simulink model "rv9level"  (R2017a)
settings: Solver=VariableStepAuto  StartTime=0.0  StopTime=0.3  MaxStep=1e-4  RelTol=1e-3
libraries: powerlib x48, simulink x4, commsynccomp2 x1, dsparch4 x1, powerlib_meascontrol x1
settings Model: Creator=Bilal Ahmed  LastModifiedBy=Bilal Ahmed

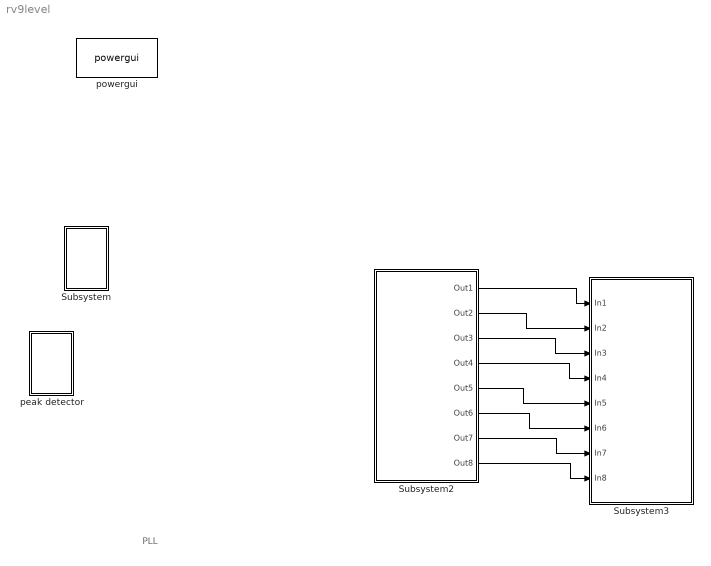
== system rv9level ==
  note: PLL
  Subsystem : Subsystem
  Subsystem2 : Subsystem
  Subsystem3 : Subsystem
  peak detector : Subsystem
  powergui : powerlib/powergui  Priority=1  SimulationMode=Continuous  SampleTime=1e-3  frequency=60  Iterations=50  frequencyindice=0  Pbase=100e6  ErrMax=1e-4  UnitsV=kV  UnitsW=MW  buscounter=0  FunctionMessages=off  echomessages=off  EnableUseOfTLC=off  CurrentSourceSwitches=off  DisableSnubberDevices=off  DisableRonSwitches=off  DisableVfSwitches=off  DisplayEquations=off  SolverType=Tustin/Backward Euler (TBE)  Interpol=off  ExternalGateDelay=off  methode=off  Ts=100  x0status=blocks  SPID=on  SwTol=0  HookPort=off  RestoreLinks=warning  ResistiveCurrentMeasurement=off  Frange=[0:2:500]  Ylog=off  Xlog=on  ShowGrid=off  save=off  variable=ZData  structure=0  ZoomFFT=off  StartTime=0.0  cycles=1  DisplayStyle=1  fundamental=60  FreqAxis=off  MaxFrequency=1000  frequencyindicesteady=1  RmsSteady=1  display=off
  wires:
  Subsystem2/3(Out3) -> Subsystem3/3(In3)
  Subsystem2/6(Out6) -> Subsystem3/6(In6)
  Subsystem2/5(Out5) -> Subsystem3/5(In5)
  Subsystem2/4(Out4) -> Subsystem3/4(In4)
  Subsystem2/2(Out2) -> Subsystem3/2(In2)
  Subsystem2/1(Out1) -> Subsystem3/1(In1)
  Subsystem2/7(Out7) -> Subsystem3/7(In7)
  Subsystem2/8(Out8) -> Subsystem3/8(In8)

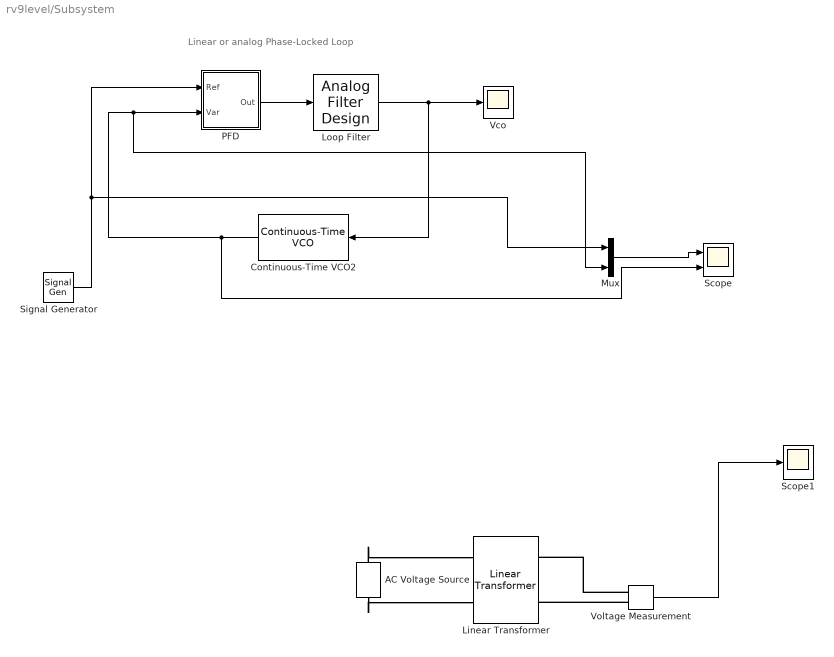
== system rv9level/Subsystem ==
  note: Linear or analog Phase-Locked Loop
  AC Voltage Source : powerlib/Electrical Sources/AC Voltage Source  Amplitude=154  Phase=0  Frequency=50  SampleTime=0  Measurements=None  BusType=PV  Pref=10e3  Qref=0  Qmin=-inf  Qmax=+inf
  Continuous-Time VCO2 : commsynccomp2/Continuous-Time VCO  Ac=2  Fc=46  Kc=8  Ph=0
      settings: SourceProductName=Communications System Toolbox  SourceProductBaseCode=CM
  Linear Transformer : powerlib/Elements/Linear Transformer  UNITS=SI  NominalPower=[ 1100 50 ]  winding1=[220 0 0]  winding2=[7 0 0]  ThreeWindings=off  winding3=[3.15e+05 7.8765e+07 26602]  RmLm=[Inf Inf]  Measurements=None  DataType=on
  Loop Filter : dsparch4/Analog Filter Design  method=Butterworth  filttype=Lowpass  N=5  Wlo=50*2*pi  Whi=80  Rp=1  Rs=180
  Mux : Mux  Inputs=2
  PFD : Subsystem
  Scope : Scope  NumInputPorts=2
  Scope1 : Scope
  Signal Generator : SignalGenerator  Amplitude=2  Frequency=2*pi*50  Units=rad/sec
  Vco : Scope
  Voltage Measurement : powerlib/Measurements/Voltage Measurement  PhasorSimulation=off  OutputType=Complex  PSBequivalent=0
  wires:
  Loop Filter/1 -> Vco/1, Continuous-Time VCO2/1
  PFD/1(Out) -> Loop Filter/1
  Mux/1 -> Scope/1
  Continuous-Time VCO2/1 -> Scope/2, Mux/2, PFD/2(Var)
  Signal Generator/1 -> Mux/1, PFD/1(Ref)
  Voltage Measurement/1 -> Scope1/1
  connections:
  AC Voltage Source/RConn1 -- Linear Transformer/LConn1
  AC Voltage Source/LConn1 -- Linear Transformer/LConn2
  Voltage Measurement/LConn1 -- Linear Transformer/RConn1
  Voltage Measurement/LConn2 -- Linear Transformer/RConn2

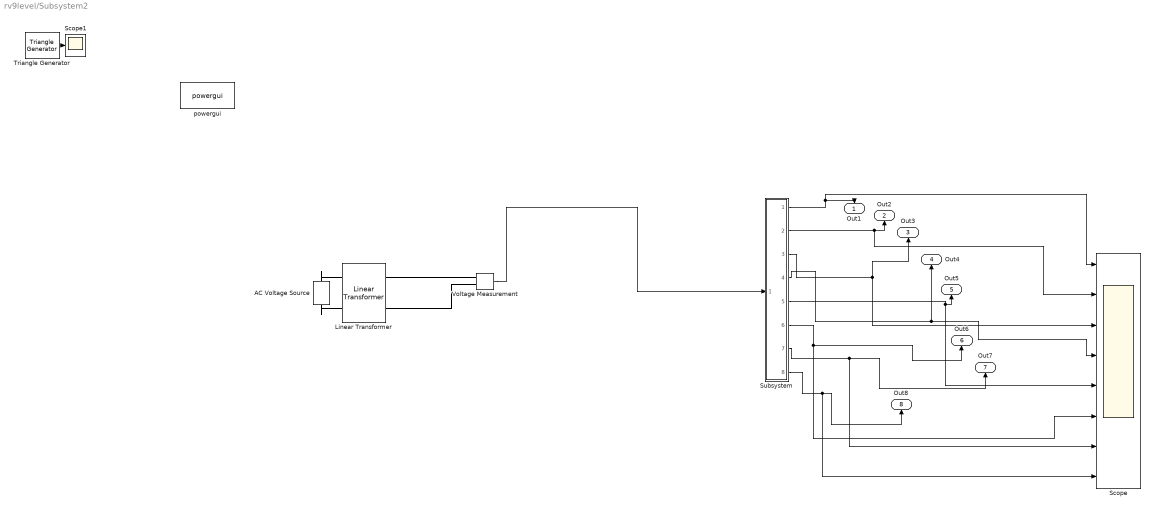
== system rv9level/Subsystem2 ==
  AC Voltage Source : powerlib/Electrical Sources/AC Voltage Source  Amplitude=220  Phase=0  Frequency=50  SampleTime=0  Measurements=None  BusType=PV  Pref=10e3  Qref=0  Qmin=-inf  Qmax=+inf
  Linear Transformer : powerlib/Elements/Linear Transformer  UNITS=pu  NominalPower=[1100 50 ]  winding1=[154 0 0]  winding2=[3.5 0 0]  ThreeWindings=off  winding3=[3.15e+05 9.68e-09 3.2267e-07]  RmLm=[Inf Inf]  Measurements=None  DataType=off
  Scope : Scope  NumInputPorts=8
  Scope1 : Scope
  Subsystem : Subsystem
  Triangle Generator : powerlib_meascontrol/Pulse & Signal Generators/Triangle Generator  Freq=1e6  Phase=0  Ts=0
  Voltage Measurement : powerlib/Measurements/Voltage Measurement  PhasorSimulation=off  OutputType=Complex  PSBequivalent=0
  powergui : powerlib/powergui  Priority=1  SimulationMode=Continuous  SampleTime=50e-6  frequency=60  Iterations=50  frequencyindice=60  Pbase=100e6  ErrMax=1e-4  UnitsV=kV  UnitsW=MW  buscounter=0  FunctionMessages=off  echomessages=off  EnableUseOfTLC=off  CurrentSourceSwitches=off  DisableSnubberDevices=off  DisableRonSwitches=off  DisableVfSwitches=off  DisplayEquations=off  SolverType=Tustin/Backward Euler (TBE)  Interpol=off  ExternalGateDelay=off  methode=off  Ts=100  x0status=blocks  SPID=on  SwTol=0  HookPort=off  RestoreLinks=warning  ResistiveCurrentMeasurement=off  Frange=[0:2:500]  Ylog=off  Xlog=on  ShowGrid=off  save=off  variable=ZData  structure=0  ZoomFFT=off  StartTime=0.0  cycles=1  DisplayStyle=1  fundamental=60  FreqAxis=off  MaxFrequency=1000  frequencyindicesteady=1  RmsSteady=1  display=off
  Out1 : Outport
  Out2 : Outport  Port=2
  Out3 : Outport  Port=3
  Out4 : Outport  Port=4
  Out5 : Outport  Port=5
  Out6 : Outport  Port=6
  Out7 : Outport  Port=7
  Out8 : Outport  Port=8
  wires:
  Voltage Measurement/1 -> Subsystem/1(In1)
  Triangle Generator/1 -> Scope1/1
  Subsystem/1(Out1) -> Scope/1, Out1/1
  Subsystem/2(Out2) -> Scope/2, Out2/1
  Subsystem/3(Out3) -> Out3/1, Scope/3
  Subsystem/6(Out4) -> Scope/6, Out6/1
  Subsystem/4(Out5) -> Scope/4, Out4/1
  Subsystem/5(Out6) -> Scope/5, Out5/1
  Subsystem/8(Out8) -> Scope/8, Out8/1
  Subsystem/7(Out7) -> Scope/7, Out7/1
  connections:
  Linear Transformer/RConn2 -- Voltage Measurement/LConn2
  AC Voltage Source/LConn1 -- Linear Transformer/LConn2
  Voltage Measurement/LConn1 -- Linear Transformer/RConn1
  AC Voltage Source/RConn1 -- Linear Transformer/LConn1

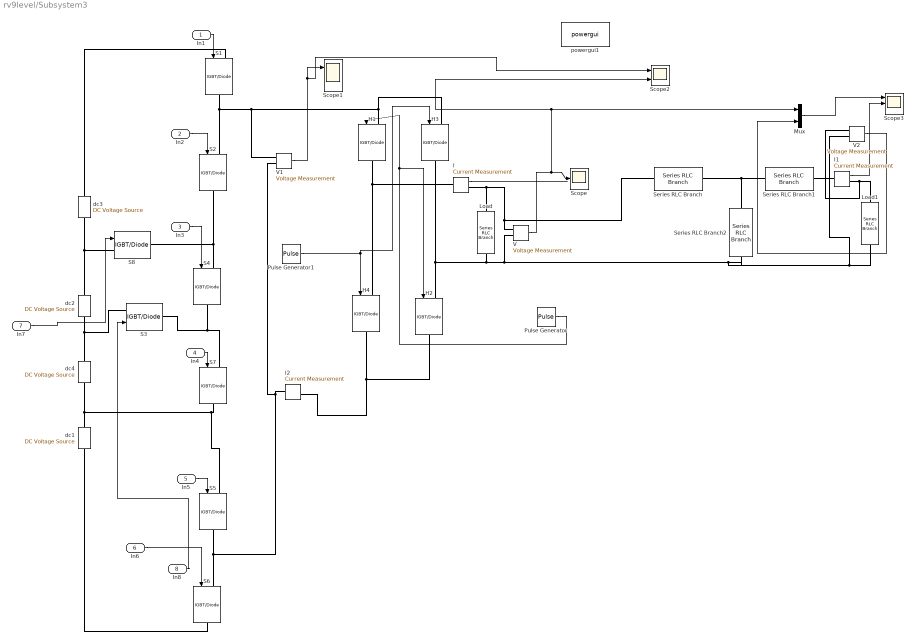
== system rv9level/Subsystem3 ==
  In1 : Inport
  In2 : Inport  Port=2
  In3 : Inport  Port=3
  In4 : Inport  Port=4
  In5 : Inport  Port=5
  In6 : Inport  Port=6
  In7 : Inport  Port=7
  In8 : Inport  Port=8
  H{1..4} (4 alike) : powerlib/Power Electronics/IGBT//Diode  Ron=1e-3  Rs=1e5  Cs=inf  Measurements=off
  I : powerlib/Measurements/Current Measurement  PhasorSimulation=off  OutputType=Complex  PSBequivalent=0
  I1 : powerlib/Measurements/Current Measurement  PhasorSimulation=off  OutputType=Complex  PSBequivalent=0
  I2 : powerlib/Measurements/Current Measurement  PhasorSimulation=off  OutputType=Complex  PSBequivalent=0
  Load : powerlib/Elements/Series RLC Branch  LConnTagsString=__new0  RConnTagsString=__new0  BranchType=R  Resistance=10  Inductance=1e-3  SetiL0=off  InitialCurrent=0  Capacitance=1e-6  Setx0=off  InitialVoltage=0  Measurements=None
  Load1 : powerlib/Elements/Series RLC Branch  LConnTagsString=__new0  RConnTagsString=__new0  BranchType=R  Resistance=10  Inductance=1e-3  SetiL0=off  InitialCurrent=0  Capacitance=1e-6  Setx0=off  InitialVoltage=0  Measurements=None
  Mux : Mux  Inputs=2
  Pulse Generator : DiscretePulseGenerator  PulseType=Time based  Period=0.02  PulseWidth=50
  Pulse Generator1 : DiscretePulseGenerator  PulseType=Time based  Period=0.02  PulseWidth=50  PhaseDelay=.01
  S{1..8} (8 alike) : powerlib/Power Electronics/IGBT//Diode  Ron=1e-3  Rs=1e5  Cs=inf  Measurements=off
  Scope : Scope
  Scope1 : Scope  NumInputPorts=2
  Scope2 : Scope  NumInputPorts=2
  Scope3 : Scope  NumInputPorts=3
  Series RLC Branch : powerlib/Elements/Series RLC Branch  LConnTagsString=__new0  RConnTagsString=__new0  BranchType=L  Resistance=1  Inductance=1e-3  SetiL0=off  InitialCurrent=0  Capacitance=1e-6  Setx0=off  InitialVoltage=0  Measurements=None
  Series RLC Branch1 : powerlib/Elements/Series RLC Branch  LConnTagsString=__new0  RConnTagsString=__new0  BranchType=L  Resistance=1  Inductance=1e-3  SetiL0=off  InitialCurrent=0  Capacitance=1e-6  Setx0=off  InitialVoltage=0  Measurements=None
  Series RLC Branch2 : powerlib/Elements/Series RLC Branch  LConnTagsString=__new0  RConnTagsString=__new0  BranchType=C  Resistance=1  Inductance=1e-3  SetiL0=off  InitialCurrent=0  Capacitance=1e-6  Setx0=off  InitialVoltage=0  Measurements=None
  V : powerlib/Measurements/Voltage Measurement  PhasorSimulation=off  OutputType=Complex  PSBequivalent=0
  V1 : powerlib/Measurements/Voltage Measurement  PhasorSimulation=off  OutputType=Complex  PSBequivalent=0
  V2 : powerlib/Measurements/Voltage Measurement  PhasorSimulation=off  OutputType=Complex  PSBequivalent=0
  dc{1..4} (4 alike) : powerlib/Electrical Sources/DC Voltage Source  Amplitude=20  Measurements=None
  powergui1 : powerlib/powergui  Priority=1  SimulationMode=Continuous  SampleTime=1e-3  frequency=60  Iterations=50  frequencyindice=0  Pbase=100e6  ErrMax=1e-4  UnitsV=kV  UnitsW=MW  buscounter=0  FunctionMessages=off  echomessages=off  EnableUseOfTLC=off  CurrentSourceSwitches=off  DisableSnubberDevices=off  DisableRonSwitches=off  DisableVfSwitches=off  DisplayEquations=off  SolverType=Tustin/Backward Euler (TBE)  Interpol=off  ExternalGateDelay=off  methode=off  Ts=100  x0status=blocks  SPID=on  SwTol=0  HookPort=off  RestoreLinks=warning  ResistiveCurrentMeasurement=off  Frange=[0:2:500]  Ylog=off  Xlog=on  ShowGrid=off  save=off  variable=ZData  structure=0  ZoomFFT=off  StartTime=0.0  cycles=1  DisplayStyle=1  fundamental=60  FreqAxis=off  MaxFrequency=1000  frequencyindicesteady=1  RmsSteady=1  display=off
  wires:
  In3/1 -> S4/1
  In6/1 -> S6/1
  In4/1 -> S7/1
  Pulse Generator1/1 -> H4/1, H3/1
  V/1 -> Mux/1, Scope2/2, Scope/1
  I/1 -> ?
  Pulse Generator/1 -> H1/1, H2/1
  In2/1 -> S2/1
  In1/1 -> S1/1
  In5/1 -> S5/1
  V1/1 -> Scope2/1, Scope1/1
  I1/1 -> Scope3/2
  V2/1 -> Mux/2
  Mux/1 -> Scope3/1
  In7/1 -> S8/1
  In8/1 -> S3/1
  connections:
  H2/RConn1 -- I2/RConn1 -- H4/RConn1
  S2/RConn1 -- S8/RConn1 -- S4/LConn1
  S4/RConn1 -- S3/RConn1 -- S7/LConn1
  dc1/LConn1 -- S6/RConn1
  I/LConn1 -- H4/LConn1 -- H1/RConn1
  H1/LConn1 -- S1/RConn1 -- S2/LConn1 -- V1/LConn1 -- H3/LConn1
  S8/LConn1 -- dc2/RConn1 -- dc3/LConn1
  H2/LConn1 -- H3/RConn1 -- Load/RConn1 -- V2/LConn2 -- Load1/RConn1 -- Series RLC Branch2/RConn1 -- V/LConn2
  dc3/RConn1 -- S1/LConn1
  Load/LConn1 -- I/RConn1 -- Series RLC Branch/LConn1 -- V/LConn1
  S5/RConn1 -- S6/LConn1 -- V1/LConn2 -- I2/LConn1
  Series RLC Branch1/LConn1 -- Series RLC Branch2/LConn1 -- Series RLC Branch/RConn1
  I1/LConn1 -- Series RLC Branch1/RConn1
  I1/RConn1 -- V2/LConn1 -- Load1/LConn1
  dc4/LConn1 -- S5/LConn1 -- S7/RConn1 -- dc1/RConn1
  dc2/LConn1 -- S3/LConn1 -- dc4/RConn1

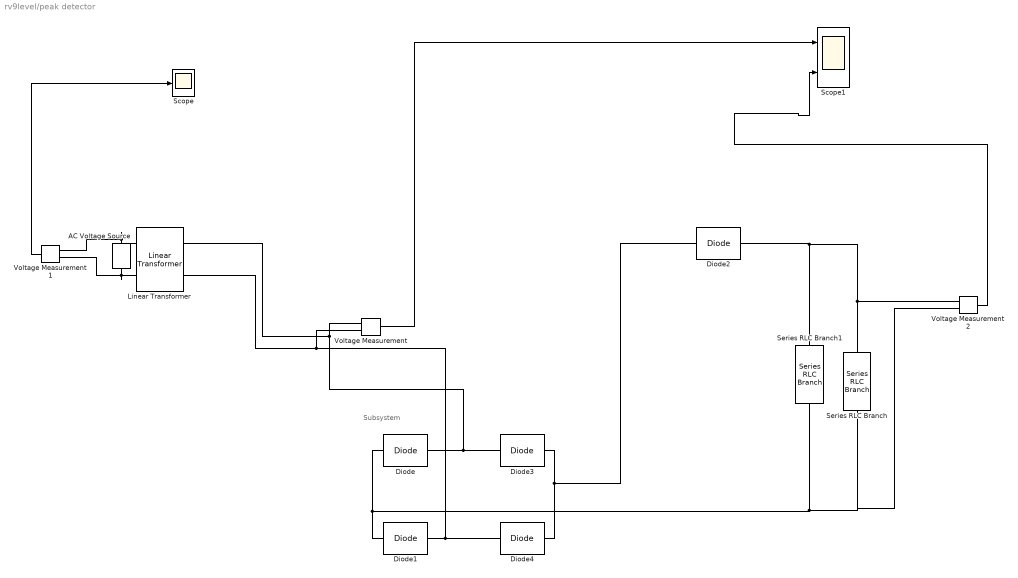
== system rv9level/peak detector ==
  note: Subsystem
  AC Voltage Source : powerlib/Electrical Sources/AC Voltage Source  Amplitude=220  Phase=0  Frequency=50  SampleTime=0  Measurements=None  BusType=PV  Pref=10e3  Qref=0  Qmin=-inf  Qmax=+inf
  Diode{,1..4} (5 alike) : powerlib/Power Electronics/Diode  Ron=0.001  Lon=0  Vf=0.03  IC=0  UseSnubber=0  Rs=500  Cs=250e-9  Measurements=off
  Linear Transformer : powerlib/Elements/Linear Transformer  UNITS=SI  NominalPower=[ 1100 50 ]  winding1=[380 0 0]  winding2=[8.641 0 0]  ThreeWindings=off  winding3=[3.15e+05 7.8765e+07 26602]  RmLm=[Inf Inf]  Measurements=None  DataType=on
  Scope : Scope
  Scope1 : Scope  NumInputPorts=2
  Series RLC Branch : powerlib/Elements/Series RLC Branch  LConnTagsString=__new0  RConnTagsString=__new0  BranchType=R  Resistance=1  Inductance=1e-3  SetiL0=off  InitialCurrent=0  Capacitance=1e-6  Setx0=off  InitialVoltage=0  Measurements=None
  Series RLC Branch1 : powerlib/Elements/Series RLC Branch  LConnTagsString=__new0  RConnTagsString=__new0  BranchType=C  Resistance=1  Inductance=1e-3  SetiL0=off  InitialCurrent=0  Capacitance=0.1  Setx0=off  InitialVoltage=0  Measurements=None
  Voltage Measurement : powerlib/Measurements/Voltage Measurement  PhasorSimulation=off  OutputType=Complex  PSBequivalent=0
  Voltage Measurement1 : powerlib/Measurements/Voltage Measurement  PhasorSimulation=off  OutputType=Complex  PSBequivalent=0
  Voltage Measurement2 : powerlib/Measurements/Voltage Measurement  PhasorSimulation=off  OutputType=Complex  PSBequivalent=0
  wires:
  Voltage Measurement1/1 -> Scope/1
  Voltage Measurement/1 -> Scope1/1
  Voltage Measurement2/1 -> Scope1/2
  connections:
  AC Voltage Source/RConn1 -- Voltage Measurement1/LConn1 -- Linear Transformer/LConn1
  AC Voltage Source/LConn1 -- Voltage Measurement1/LConn2 -- Linear Transformer/LConn2
  Diode1/RConn1 -- Diode4/LConn1 -- Linear Transformer/RConn2 -- Voltage Measurement/LConn2
  Diode4/RConn1 -- Diode2/LConn1 -- Diode3/RConn1
  Voltage Measurement/LConn1 -- Linear Transformer/RConn1 -- Diode/RConn1 -- Diode3/LConn1
  Series RLC Branch/RConn1 -- Series RLC Branch1/LConn1 -- Diode2/RConn1 -- Voltage Measurement2/LConn1
  Diode/LConn1 -- Voltage Measurement2/LConn2 -- Series RLC Branch/LConn1 -- Series RLC Branch1/RConn1 -- Diode1/LConn1

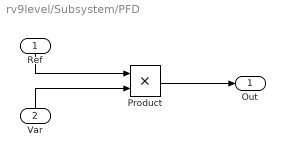
== system rv9level/Subsystem/PFD ==
  Ref : Inport
  Var : Inport  Port=2
  Product : Product  RndMeth=Zero
  Out : Outport
  wires:
  Ref/1 -> Product/1
  Var/1 -> Product/2
  Product/1 -> Out/1

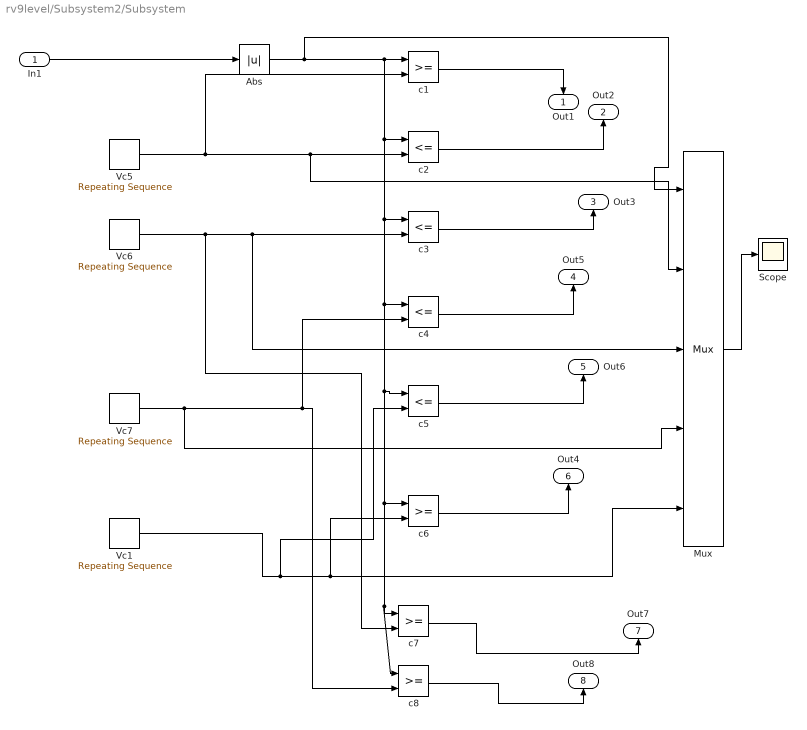
== system rv9level/Subsystem2/Subsystem ==
  In1 : Inport
  Abs : Abs
  Mux : Mux  Inputs=5
  Scope : Scope
  Vc1 : simulink/Sources/Repeating Sequence  rep_seq_t=[0 0.00001/2 0.00001]  rep_seq_y=[0 1.25 0]
  Vc5 : simulink/Sources/Repeating Sequence  rep_seq_t=[0 0.00001/2 0.00001]  rep_seq_y=[3.75 5.00 3.75]
  Vc6 : simulink/Sources/Repeating Sequence  rep_seq_t=[0 0.00001/2 0.00001]  rep_seq_y=[2.50 3.75 2.50]
  Vc7 : simulink/Sources/Repeating Sequence  rep_seq_t=[0 0.00001/2 0.00001]  rep_seq_y=[1.25 2.50 1.25]
  c{1,6..8} (4 alike) : RelationalOperator  OutDataTypeStr=boolean  RndMeth=Nearest
  c{2..5} (4 alike) : RelationalOperator  Operator=<=  OutDataTypeStr=boolean  RndMeth=Nearest
  Out1 : Outport
  Out2 : Outport  Port=2
  Out3 : Outport  Port=3
  Out5 : Outport  Port=4
  Out6 : Outport  Port=5
  Out4 : Outport  Port=6
  Out7 : Outport  Port=7
  Out8 : Outport  Port=8
  wires:
  c5/1 -> Out6/1
  c6/1 -> Out4/1
  c4/1 -> Out5/1
  c2/1 -> Out2/1
  c1/1 -> Out1/1
  Vc7/1 -> Mux/4, c8/2, c4/2
  Vc5/1 -> c1/2, Mux/2, c2/2
  Vc6/1 -> c7/2, Mux/3, c3/2
  Mux/1 -> Scope/1
  c3/1 -> Out3/1
  Abs/1 -> Mux/1, c2/1, c5/1, c6/1, c8/1, c7/1, c4/1, c3/1, c1/1
  In1/1 -> Abs/1
  Vc1/1 -> c5/2, c6/2, Mux/5
  c7/1 -> Out7/1
  c8/1 -> Out8/1
